simulink model "model5Matlab"  (R2015a)
settings: Solver=ode45  SolverMode=SingleTasking  StartTime=0.0  StopTime=500  RelTol=1e-3
values from neighbouring files (symbols this model uses):
  A_d = [0.996954078594 -0.0607605694933 0 0 0 0.0992753993526 0.98452749568 0 0 0 0 0 ... (25 elements, 5x5)]    [A_d.mat]
  B_d = [0 0 8.38564521491e-06 0.000153104191579 0]    [data_matrix_B_d.mat]
  C_d = [0 1 1 0 0]    [data_matrix_C_d.mat]    (also in script_boat.m = C)
  E_d = [2.39991691766e-05  0; 0.00047873959707  0; 0  -2.92394580282e-07; 0  -8.38564521491e-06; 0  0.1]    [E_d.mat]
  Kpd = 0.7612    [script_boat.m]
  P_0 = [1 0 0 0 0 0 0.013 0 0 0 0 0 ... (25 elements, 5x5)]    [P_0.mat]    (also in script_boat.m = [1 0 0 0 0; 0 0.013 0 0 0; 0 0 pi^2 0 0; 0 0 0 1 0; 0 0 0 0 )
  Q = [30  0; 0  1e-05]    [data_matrix_Q.mat]    (also in script_boat.m = [30 0; 0 10e-6])
  R = 6.02263276801e-06    [data_matrix_R.mat]    (also in script_boat.m = m_var/Ts)
  Td = T    [script_boat.m]
  Tf = 8.5    [script_boat.m]
  Ts = 0.1    [script_boat.m]
libraries: simulink x2
settings Model: Creator=markh  LastModifiedBy=mortejan
settings OptimizationCC: BlockReduction=off  BooleanDataType=off
settings DebuggingCC: SaveWithParameterizedLinksMsg=none  UnderspecifiedInitializationDetection=Classic  MergeDetectMultiDrivingBlocksExec=none  SignalResolutionControl=TryResolveAllWithWarning
settings HardwareCC: TargetUnknown=on

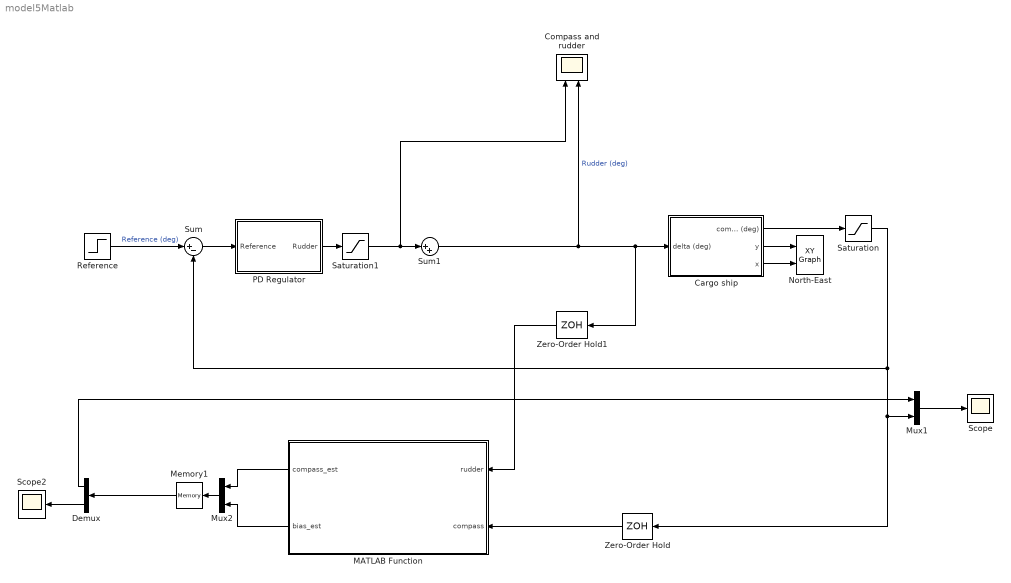
== system model5Matlab ==
  Cargo ship : Subsystem  mask(Simple shipmodel for a cargo ship){noise=on, current=on, logic=off}
      mask prompts: noise "measurement noise"; logic "waves"
      mask help:
      | Measurement noise:
      | 	checked = noise on
      | 	unchecked = noise off
      |
      | Current:
      | 	checked = current on
      | 	unchecked = current off
      |
      | Waves:
      | 	checked = waves on
      | 	unchecked = waves off
      |
      | Author: Jørgen Spjøtvold, 9/10-2003
      | TTK 4115 Linear system theory.
      | Modified by Jostein Bakkeheim 26/10-2006
  Compass and rudder : Scope  NumInputPorts=2
      settings: ShowLegends=on  TimeRange=500  YMin=-1~-1  YMax=1.25~1.25  SaveName=w2_smooth1  MaxDataPoints=2000
  Demux : Demux  Outputs=2
  MATLAB Function : MATLAB Function  TreatAsAtomicUnit=on
  Memory1 : Memory
  Mux1 : Mux  Inputs=2
  Mux2 : Mux  Inputs=2
  North-East : simulink/Sinks/XY Graph  xmin=-5000  xmax=5000  ymin=-5000  ymax=5000  st=-1
  PD Regulator : Subsystem
  Reference : Step  After=30  SampleTime=0
  Saturation : Saturate  UpperLimit=35  LowerLimit=-35
  Saturation1 : Saturate  UpperLimit=45  LowerLimit=-45
  Scope : Scope
      settings: ShowLegends=on  YMin=25.35  YMax=26.15
  Scope2 : Scope
      settings: ShowLegends=on  YMin=-175  YMax=0  SaveName=ScopeData2
  Sum : Sum  Inputs=|+-
  Sum1 : Sum  Inputs=|++
  Zero-Order Hold : ZeroOrderHold  SampleTime=Ts
  Zero-Order Hold1 : ZeroOrderHold  SampleTime=Ts
  wires:
  Cargo ship/3(x) -> North-East/2
  Cargo ship/2(y) -> North-East/1
  Reference/1 -> Sum/1  "Reference (deg)"
  Sum/1 -> PD Regulator/1(Reference)
  Sum1/1 -> Zero-Order Hold1/1, Cargo ship/1(delta (deg)), Compass and rudder/2  "Rudder (deg)"
  Cargo ship/1(compass (deg)) -> Saturation/1
  PD Regulator/1(Rudder) -> Saturation1/1
  MATLAB Function/1(compass_est) -> Mux2/1
  Zero-Order Hold/1 -> MATLAB Function/2(compass)
  MATLAB Function/2(bias_est) -> Mux2/2
  Mux1/1 -> Scope/1
  Mux2/1 -> Memory1/1
  Saturation1/1 -> Compass and rudder/1, Sum1/1
  Demux/1 -> Mux1/1
  Demux/2 -> Scope2/1
  Memory1/1 -> Demux/1
  Saturation/1 -> Sum/2, Mux1/2, Zero-Order Hold/1
  Zero-Order Hold1/1 -> MATLAB Function/1(rudder)

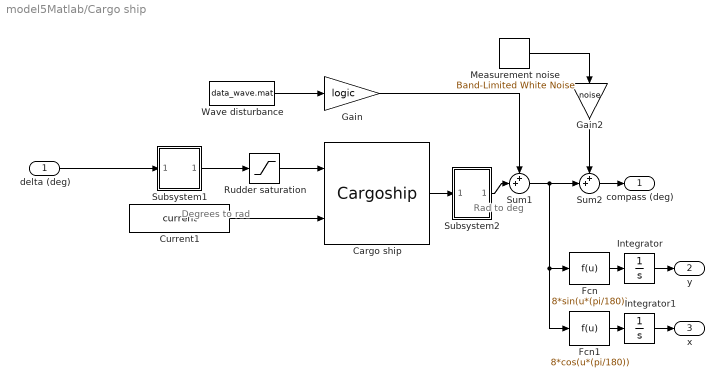
== system model5Matlab/Cargo ship ==
  note: Degrees to rad
  note: Rad to deg
  delta (deg) : Inport
  Cargo ship : S-Function  FunctionName=Cargoship  mask(Cargo ship){}
      mask help:
      | S-function which simulates a cargo ship.
      |
      | Author: Jørgen Spjøtvold
      | 20.10-2003
      | Modified by Jostein Bakkeheim 27.10.2006
  Current1 : Constant  Value=current
  Fcn : Fcn  Expr=8*sin(u*(pi/180))
  Fcn1 : Fcn  Expr=8*cos(u*(pi/180))
  Gain : Gain  Gain=logic  SaturateOnIntegerOverflow=on  OutDataTypeStr=Inherit: Same as input  ParamDataTypeStr=Inherit: Same as input
  Gain2 : Gain  Gain=noise  SaturateOnIntegerOverflow=on  OutDataTypeStr=Inherit: Same as input  ParamDataTypeStr=Inherit: Same as input
  Integrator : Integrator
  Integrator1 : Integrator
  Measurement noise : simulink/Sources/Band-Limited White Noise  Cov=[0.001]  Ts=.5  seed=[23341]
  Rudder saturation : Saturate  UpperLimit=45*(pi/180)  LowerLimit=-45*(pi/180)
  Subsystem1 : Subsystem  mask(degrees to radians){}
      mask help: Converts degrees to radians
      mask Display: fprintf('D2R');
  Subsystem2 : Subsystem  mask(radians to degrees){}
      mask help: Converts radians to degrees
      mask Display: fprintf('R2D');
  Sum1 : Sum  Inputs=++|  SaturateOnIntegerOverflow=on
  Sum2 : Sum  Inputs=++|  SaturateOnIntegerOverflow=on
  Wave disturbance : FromFile  FileName=data_wave.mat  SampleTime=0
  compass (deg) : Outport
  y : Outport  Port=2
  x : Outport  Port=3
  wires:
  delta (deg)/1 -> Subsystem1/1(In1)
  Fcn/1 -> Integrator/1
  Integrator/1 -> y/1
  Fcn1/1 -> Integrator1/1
  Integrator1/1 -> x/1
  Wave disturbance/1 -> Gain/1
  Subsystem2/1(Out1) -> Sum1/2
  Gain/1 -> Sum1/1
  Sum1/1 -> Fcn/1, Fcn1/1, Sum2/2
  Cargo ship/1 -> Subsystem2/1(In1)
  Subsystem1/1(Out1) -> Rudder saturation/1
  Rudder saturation/1 -> Cargo ship/1
  Sum2/1 -> compass (deg)/1
  Measurement noise/1 -> Gain2/1
  Gain2/1 -> Sum2/1
  Current1/1 -> Cargo ship/2

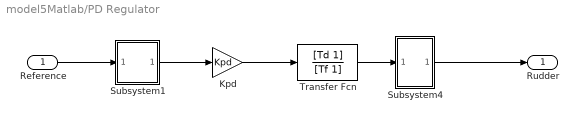
== system model5Matlab/PD Regulator ==
  Reference : Inport
  Kpd : Gain  Gain=Kpd
  Subsystem1 : Subsystem  mask(degrees to radians){}
      mask help: Converts degrees to radians
      mask Display: fprintf('D2R');
  Subsystem4 : Subsystem  mask(radians to degrees){}
      mask help: Converts radians to degrees
      mask Display: fprintf('R2D');
  Transfer Fcn : TransferFcn  Numerator=[Td 1]  Denominator=[Tf 1]
  Rudder : Outport
  wires:
  Reference/1 -> Subsystem1/1(In1)
  Kpd/1 -> Transfer Fcn/1
  Transfer Fcn/1 -> Subsystem4/1(In1)
  Subsystem4/1(Out1) -> Rudder/1
  Subsystem1/1(Out1) -> Kpd/1

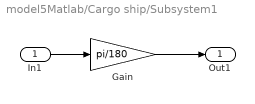
== system model5Matlab/Cargo ship/Subsystem1 ==
  In1 : Inport
  Gain : Gain  Gain=pi/180  SaturateOnIntegerOverflow=on  OutDataTypeStr=Inherit: Same as input  ParamDataTypeStr=Inherit: Same as input
  Out1 : Outport
  wires:
  Gain/1 -> Out1/1
  In1/1 -> Gain/1

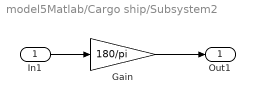
== system model5Matlab/Cargo ship/Subsystem2 ==
  In1 : Inport
  Gain : Gain  Gain=180/pi  SaturateOnIntegerOverflow=on  OutDataTypeStr=Inherit: Same as input  ParamDataTypeStr=Inherit: Same as input
  Out1 : Outport
  wires:
  Gain/1 -> Out1/1
  In1/1 -> Gain/1

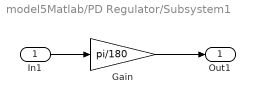
== system model5Matlab/PD Regulator/Subsystem1 ==
  In1 : Inport
  Gain : Gain  Gain=pi/180  SaturateOnIntegerOverflow=on  OutDataTypeStr=Inherit: Same as input  ParamDataTypeStr=Inherit: Same as input
  Out1 : Outport
  wires:
  Gain/1 -> Out1/1
  In1/1 -> Gain/1

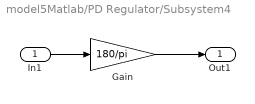
== system model5Matlab/PD Regulator/Subsystem4 ==
  In1 : Inport
  Gain : Gain  Gain=180/pi  SaturateOnIntegerOverflow=on  OutDataTypeStr=Inherit: Same as input  ParamDataTypeStr=Inherit: Same as input
  Out1 : Outport
  wires:
  Gain/1 -> Out1/1
  In1/1 -> Gain/1

== matlab function model5Matlab/MATLAB Function ==
  data: rudder input; compass input; compass_est output; bias_est output; A_d parameter; B_d parameter; C_d parameter; E_d parameter; R parameter; Q parameter; P_0 parameter

function [compass_est, bias_est] = Kalman(rudder,compass,A_d,B_d,C_d,E_d,R,Q,P_0)
%#codegen

persistent init_flag x_nextPri P_nextPri

if isempty(init_flag)
    init_flag = 1;
    x_nextPri = [0;0;0;0;0];
    P_nextPri = P_0;
end

I = eye(5);

P_pri = P_nextPri;
x_pri = x_nextPri;

K_k =  P_pri*C_d'*inv(C_d*P_pri*C_d'+R);

x_post = x_pri + K_k*(compass-C_d*x_pri);

P_k = (I-K_k*C_d)*P_pri*(I-K_k*C_d)'+K_k*R*K_k';

x_nextPri = A_d*x_post + B_d*rudder;

P_nextPri = A_d*P_k*A_d'+E_d*Q*E_d';

compass_est = x_post(3);
bias_est = x_post(5);
